simulink model "sensores_no_ideales_en_SS"  (R2023b)
settings: Solver=VariableStepAuto  StartTime=0.0  StopTime=10.0  RelTol=1e-3
undefined symbols (not defined in the file or in its folder): A_iabc, A_pos, A_T, B_iabc, B_pos, B_T, C_iabc, C_pos, C_T, D_iabc, D_pos, D_T
settings Model: Creator=Pc  LastModifiedBy=Pc

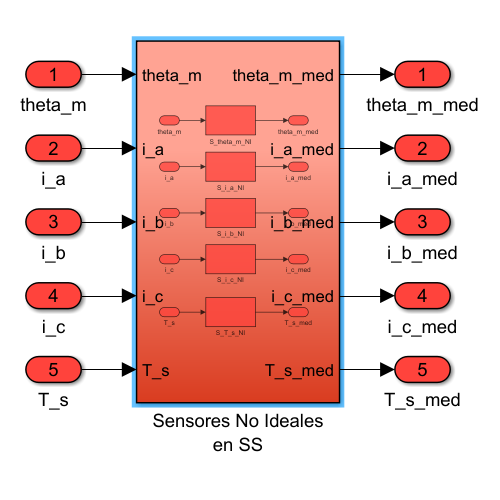
[thumbnail: Simulink's stored preview of the top-level diagram]
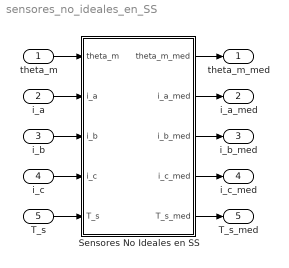
== system sensores_no_ideales_en_SS ==
  theta_m : Inport
  i_a : Inport  Port=2
  i_b : Inport  Port=3
  i_c : Inport  Port=4
  T_s : Inport  Port=5
  Sensores No Ideales en SS : Subsystem
  theta_m_med : Outport
  i_a_med : Outport  Port=2
  i_b_med : Outport  Port=3
  i_c_med : Outport  Port=4
  T_s_med : Outport  Port=5
  wires:
  theta_m/1 -> Sensores No Ideales en SS/1(theta_m)
  i_a/1 -> Sensores No Ideales en SS/2(i_a)
  i_b/1 -> Sensores No Ideales en SS/3(i_b)
  i_c/1 -> Sensores No Ideales en SS/4(i_c)
  T_s/1 -> Sensores No Ideales en SS/5(T_s)
  Sensores No Ideales en SS/1(theta_m_med) -> theta_m_med/1
  Sensores No Ideales en SS/2(i_a_med) -> i_a_med/1
  Sensores No Ideales en SS/3(i_b_med) -> i_b_med/1
  Sensores No Ideales en SS/4(i_c_med) -> i_c_med/1
  Sensores No Ideales en SS/5(T_s_med) -> T_s_med/1

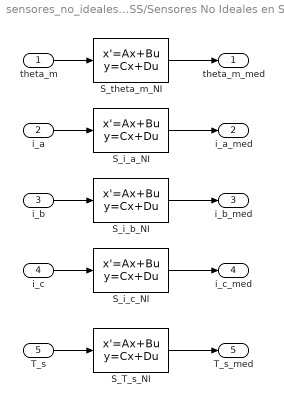
== system sensores_no_ideales_en_SS/Sensores No Ideales en SS ==
  theta_m : Inport
  i_a : Inport  Port=2
  i_b : Inport  Port=3
  i_c : Inport  Port=4
  T_s : Inport  Port=5
  S_T_s_NI : StateSpace  A=A_T  B=B_T  C=C_T  D=D_T  InitialCondition=0
  S_i_a_NI : StateSpace  A=A_iabc  B=B_iabc  C=C_iabc  D=D_iabc  InitialCondition=0
  S_i_b_NI : StateSpace  A=A_iabc  B=B_iabc  C=C_iabc  D=D_iabc  InitialCondition=0
  S_i_c_NI : StateSpace  A=A_iabc  B=B_iabc  C=C_iabc  D=D_iabc  InitialCondition=0
  S_theta_m_NI : StateSpace  A=A_pos  B=B_pos  C=C_pos  D=D_pos  InitialCondition=0
  theta_m_med : Outport
  i_a_med : Outport  Port=2
  i_b_med : Outport  Port=3
  i_c_med : Outport  Port=4
  T_s_med : Outport  Port=5
  wires:
  S_i_b_NI/1 -> i_b_med/1
  i_b/1 -> S_i_b_NI/1
  T_s/1 -> S_T_s_NI/1
  i_c/1 -> S_i_c_NI/1
  S_i_c_NI/1 -> i_c_med/1
  S_T_s_NI/1 -> T_s_med/1
  i_a/1 -> S_i_a_NI/1
  S_theta_m_NI/1 -> theta_m_med/1
  theta_m/1 -> S_theta_m_NI/1
  S_i_a_NI/1 -> i_a_med/1
